simulink model "Loop_detailed_model_v12_bipolar"  (R2013a)
settings: Solver=ode3  SolverMode=SingleTasking  StartTime=0.0  StopTime=8e-3  FixedStep=FS/50  MaxStep=1e-4  RelTol=1e-3
InitFcn:
  | %%%%%%  set scope time range
  | T_STOP=str2num(get_param(gcs,'StopTime'));
  | if numel(T_STOP) > 1
  |    T_STOP=T_STOP(2);
  | else
  |    T_STOP=T_STOP(1);
  | end
  | T_STOP=num2str(T_STOP);
  | 
  | %%%%%%  set scope time range in system @init_callback_fct
  | T_STOP=num2str(str2num(get_param(gcs,'StopTime')));
  | 
  | childs = allchild(0);
  | sol=strfind(upper(get(allchild(0),'Tag')),'VIEWER_PARAMETERS');
  | 
  | if iscell(sol)
  |    ind=find(~cellfun(@isempty, strfind(upper(get(allchild(0),'Tag')),'VIEWER_PARAMETERS')));
  | else
  |    ind=sol;
  | end
  | %ind=find(~cellfun(@isempty, {strfind(upper(get(allchild(0),'Tag')),'VIEWER_PARAMETERS'),[]}))
  | if ~isempty(ind)
  |    for k=1:length(childs(ind))
  |       set_param(getfield(get(childs(ind(k)),'UserData'),'block'),'TimeRange', T_STOP);
  | %      get_param(getfield(get(childs(ind(k)),'UserData'),'block'),'TimeRange');
  | %    set_param(getfield(get(childs(ind),'UserData'),'block'),'TimeRange',T_STOP);
  | %    get_param(getfield(get(childs(ind),'UserData'),'block'),'TimeRange');
  |    end
  | else
  |     warning(sprintf('VIEWER_PARAMETERS object not found\nOpen the config dialog by hand for the first sim start'))
  | end
values from neighbouring files (symbols this model uses):
  FS = 5e-6    (= 5e-06)    [GalvoModel_v4_sys.m]    (also in GalvoModel_v6_sys.m = 5e-05; Galvo_process_analyze.m = 0.0001)
  Lc = 170e-6    (= 0.00017)    [GalvoModel_v6_sys.m]    (also in Galvo_process_analyze.m)
  Rc = 1.5    [GalvoModel_v6_sys.m]    (also in Galvo_process_analyze.m; frequenzgang_nichtinvert_opamp_koblitz_eas.m = 1)
  Rsh = 0.003    [GalvoModel_v6_sys.m]    (also in Galvo_sys_proto_v13_OFFSETS_MODEL_PT1B_proc.m = 0.075; frequenzgang_nichtinvert_opamp_koblitz_eas.m = 0.015)
  T1 = R1*C1    (= 0.000264)    [GalvoModel_v6_sys.m]
libraries: simulink x4
settings Model: BufferReuse=off  Creator=mainster  LastModifiedBy=mainster
settings SolverCC: AutoInsertRateTranBlk=on
settings OptimizationCC: InlineParams=on  BufferReuse=off
settings DebuggingCC: InitInArrayFormatMsg=none
settings HardwareCC: ProdLargestAtomicInteger=Long  ProdLargestAtomicFloat=Double  ProdEndianess=LittleEndian  ProdHWDeviceType=ARM Compatible->ARM Cortex

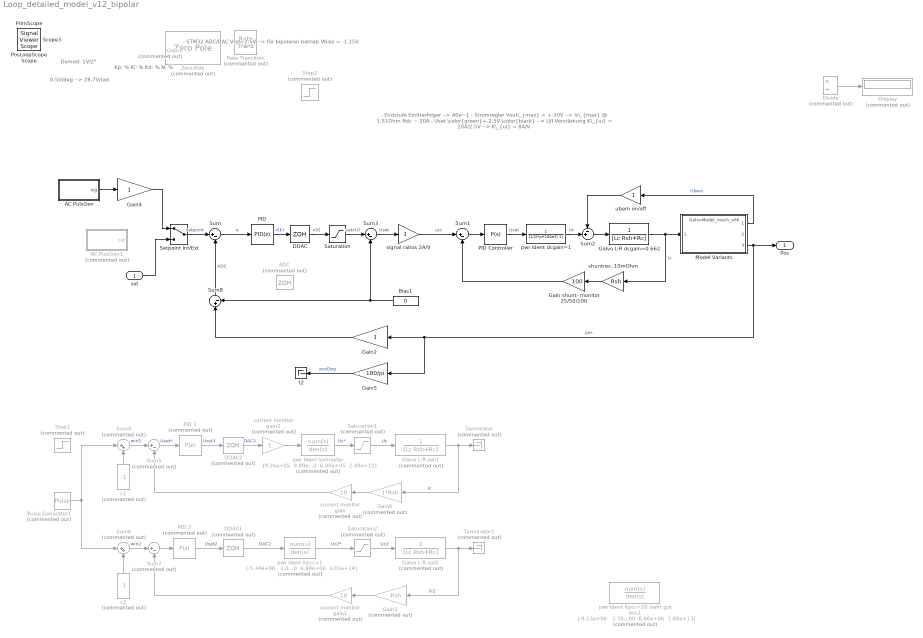
== system Loop_detailed_model_v12_bipolar ==
  note: - Endstufe Emitterfolger --> A0e~1
      | - Stromregler Vout\_{max} = +-30V
      |       --> Ic\_{max} @ 1.51Ohm Rdc ~ 20A
      | - Uset \color{green}+-2.5V \color{black}
      |       --> U/I Verstärkung K\_{ui} = 20A/2.5V
      |       --> K\_{ui} = 8A/V
  note: - STM32 ADC/DAC Vref=2.5V
      | --> für bipolaren betrieb Vbias = -1.25V
  note: Kp: % Ki: % Kd: % N: %
  note: 0.5V/deg --> 28.7V/rad
  note: Demod:
      | 1V/2°
  set : Inport
  AC PulsGen : Subsystem  mask{sigp=10, sigpp=0, offs=0}
      mask prompts: sigp "Insert signal peak"; sigpp "or signal peak-to-peak"; offs "Insert DC offset"
      mask TypeOptions sigp: PulsGen/Amplitude
      mask Callback sigp:
      | %sigp=get_param([gcb '/PulsGen'],'Amplitude')
      | %SigVal=2*sigp
      mask TypeOptions offs: offset/Value
      mask Display:
      | %str=sprintf('%s',get(gcbh,'ModelName'));
      | port_label('output', 1, '','texmode','off')
      | %text(.05,.98,['{\fontsize{12}\it\bf' strrep(str,'_',' ') '}'],'horizontalAlignment','left','verticalAlignment','top','texmode','on')
      | %text(.5,0.95,['{\fontsize{8}A_{peak}=}'],'horizontalAlignment','center','verticalAlignment','top','texmode','on')
      | disp(sprintf('Up=%.3g\nDC=%.3g',sigp, offs))
      | %disp(['Upp=' sigpp])%, offs))
      | %sprintf('sigpp==%s',sigpp)
      | %text(.15,.05,['{\fontsize{10}\itmechanics}'],'horizontalAlignment','left','verticalAlignment','bottom','texmode','on')
  AC PulsGen1 : Subsystem  Commented=on  mask{sigp=1, sigpp=0, offs=0}
      mask prompts: sigp "Insert signal peak"; sigpp "or signal peak-to-peak"; offs "Insert DC offset"
      mask TypeOptions sigp: PulsGen/Amplitude
      mask Callback sigp:
      | %sigp=get_param([gcb '/PulsGen'],'Amplitude')
      | %SigVal=2*sigp
      mask TypeOptions offs: offset/Value
      mask Display:
      | %str=sprintf('%s',get(gcbh,'ModelName'));
      | port_label('output', 1, '','texmode','off')
      | %text(.05,.98,['{\fontsize{12}\it\bf' strrep(str,'_',' ') '}'],'horizontalAlignment','left','verticalAlignment','top','texmode','on')
      | %text(.5,0.95,['{\fontsize{8}A_{peak}=}'],'horizontalAlignment','center','verticalAlignment','top','texmode','on')
      | disp(sprintf('Up=%.3g\nDC=%.3g',sigp, offs))
      | %disp(['Upp=' sigpp])%, offs))
      | %sprintf('sigpp==%s',sigpp)
      | %text(.15,.05,['{\fontsize{10}\itmechanics}'],'horizontalAlignment','left','verticalAlignment','bottom','texmode','on')
  ADC : ZeroOrderHold  Commented=on  SampleTime=FS
  Bias1 : Constant  Value=0  OutDataTypeStr=double  SampleTime=0
  DDAC : ZeroOrderHold  SampleTime=FS
      settings: AttributesFormatString=%<SampleTime>
  DDAC1 : ZeroOrderHold  Commented=on  SampleTime=FS
      settings: AttributesFormatString=%<SampleTime>
  DDAC2 : ZeroOrderHold  Commented=on  SampleTime=FS
      settings: AttributesFormatString=%<SampleTime>
  Display : Display  Commented=on
  Divide : Product  Commented=on  Inputs=*/
  Gain shunt- monitor 25/50/100 : Gain  Gain=100
  Gain1 : Gain  Commented=on  Gain=2
  Gain2 : Gain
  Gain3 : Gain  Commented=on  Gain=Rsh
  Gain4 : Gain  SampleTime=FS
  Gain5 : Gain  Gain=180/pi
  Gain6 : Gain  Commented=on  Gain=1*Rsh
  Galvo L-R dcgain=0.662 : TransferFcn  Numerator=1  Denominator=[Lc Rsh+Rc]
  Galvo L-R zeil1 : TransferFcn  Commented=on  Numerator=1  Denominator=[Lc Rsh+Rc]
  Galvo L-R zeil2 : TransferFcn  Commented=on  Numerator=1  Denominator=[Lc Rsh+Rc]
  Model Variants : ModelReference  ModelNameDialog=GalvoModel_mech_v60.slx  SimulationMode=Normal  ModelReferenceVersion=1.68  CopyOfModelName=GalvoModel_mech_v60.slx  DefaultDataLogging=on
      settings: AttributesFormatString=%<ActiveVariant>
  "PID " : simulink/Continuous/PID Controller  Controller=PID  TimeDomain=Discrete-time  SampleTime=FS  IntegratorMethod=Forward Euler  FilterMethod=Forward Euler  Form=Ideal  P=0.0159567680889438  I=1.35343300474195  D=0.0839511753460528  N=253.181387711443  InitialConditionSource=internal  InitialConditionForIntegrator=0  InitialConditionForFilter=0  ExternalReset=none  LimitOutput=off  UpperSaturationLimit=1.25  LowerSaturationLimit=-1.25  LinearizeAsGain=on  AntiWindupMode=clamping  Kb=1  TrackingMode=off  Kt=1  PParamMin=[]  PParamMax=[]  IParamMin=[]  IParamMax=[]  DParamMin=[]  DParamMax=[]  NParamMin=[]  NParamMax=[]  KbParamMin=[]  KbParamMax=[]  KtParamMin=[]  KtParamMax=[]  POutMin=[]  POutMax=[]  IOutMin=[]  IOutMax=[]  DOutMin=[]  DOutMax=[]  NOutMin=[]  NOutMax=[]  KbOutMin=[]  KbOutMax=[]  KtOutMin=[]  KtOutMax=[]  IntegratorOutMin=[]  IntegratorOutMax=[]  FilterOutMin=[]  FilterOutMax=[]  SumOutMin=[]  SumOutMax=[]  SumI1OutMin=[]  SumI1OutMax=[]  SumI2OutMin=[]  SumI2OutMax=[]  SumI3OutMin=[]  SumI3OutMax=[]  SumDOutMin=[]  SumDOutMax=[]  SaturationOutMin=[]  SaturationOutMax=[]  IntegratorContinuousStateAttributes=''  IntegratorStateMustResolveToSignalObject=off  IntegratorRTWStateStorageClass=Auto  FilterContinuousStateAttributes=''  FilterStateMustResolveToSignalObject=off  FilterRTWStateStorageClass=Auto
      settings: AttributesFormatString=UpLim=%<UpperSaturationLimit>\nLoLim=%<LowerSaturationLimit>\nKp=%<P>
  PID 1 : simulink/Continuous/PID Controller  Commented=on  Controller=P  TimeDomain=Discrete-time  SampleTime=FS  IntegratorMethod=Forward Euler  FilterMethod=Forward Euler  Form=Parallel  P=25.2263389172728  I=3745.38790742202  D=9.0248898483108e-05  N=10930.7783722874  InitialConditionSource=internal  InitialConditionForIntegrator=0  InitialConditionForFilter=0  ExternalReset=none  LimitOutput=off  UpperSaturationLimit=1.25  LowerSaturationLimit=-1.25  LinearizeAsGain=on  AntiWindupMode=clamping  Kb=1  TrackingMode=off  Kt=1  PParamMin=[]  PParamMax=[]  IParamMin=[]  IParamMax=[]  DParamMin=[]  DParamMax=[]  NParamMin=[]  NParamMax=[]  KbParamMin=[]  KbParamMax=[]  KtParamMin=[]  KtParamMax=[]  POutMin=[]  POutMax=[]  IOutMin=[]  IOutMax=[]  DOutMin=[]  DOutMax=[]  NOutMin=[]  NOutMax=[]  KbOutMin=[]  KbOutMax=[]  KtOutMin=[]  KtOutMax=[]  IntegratorOutMin=[]  IntegratorOutMax=[]  FilterOutMin=[]  FilterOutMax=[]  SumOutMin=[]  SumOutMax=[]  SumI1OutMin=[]  SumI1OutMax=[]  SumI2OutMin=[]  SumI2OutMax=[]  SumI3OutMin=[]  SumI3OutMax=[]  SumDOutMin=[]  SumDOutMax=[]  SaturationOutMin=[]  SaturationOutMax=[]  IntegratorContinuousStateAttributes=''  IntegratorStateMustResolveToSignalObject=off  IntegratorRTWStateStorageClass=Auto  FilterContinuousStateAttributes=''  FilterStateMustResolveToSignalObject=off  FilterRTWStateStorageClass=Auto
  PID 2 : simulink/Continuous/PID Controller  Commented=on  Controller=P  TimeDomain=Discrete-time  SampleTime=FS  IntegratorMethod=Forward Euler  FilterMethod=Forward Euler  Form=Parallel  P=9.78763876336799  I=3745.38790742202  D=9.0248898483108e-05  N=10930.7783722874  InitialConditionSource=internal  InitialConditionForIntegrator=0  InitialConditionForFilter=0  ExternalReset=none  LimitOutput=off  UpperSaturationLimit=1.25  LowerSaturationLimit=-1.25  LinearizeAsGain=on  AntiWindupMode=clamping  Kb=1  TrackingMode=off  Kt=1  PParamMin=[]  PParamMax=[]  IParamMin=[]  IParamMax=[]  DParamMin=[]  DParamMax=[]  NParamMin=[]  NParamMax=[]  KbParamMin=[]  KbParamMax=[]  KtParamMin=[]  KtParamMax=[]  POutMin=[]  POutMax=[]  IOutMin=[]  IOutMax=[]  DOutMin=[]  DOutMax=[]  NOutMin=[]  NOutMax=[]  KbOutMin=[]  KbOutMax=[]  KtOutMin=[]  KtOutMax=[]  IntegratorOutMin=[]  IntegratorOutMax=[]  FilterOutMin=[]  FilterOutMax=[]  SumOutMin=[]  SumOutMax=[]  SumI1OutMin=[]  SumI1OutMax=[]  SumI2OutMin=[]  SumI2OutMax=[]  SumI3OutMin=[]  SumI3OutMax=[]  SumDOutMin=[]  SumDOutMax=[]  SaturationOutMin=[]  SaturationOutMax=[]  IntegratorContinuousStateAttributes=''  IntegratorStateMustResolveToSignalObject=off  IntegratorRTWStateStorageClass=Auto  FilterContinuousStateAttributes=''  FilterStateMustResolveToSignalObject=off  FilterRTWStateStorageClass=Auto
  PID Controller : simulink/Continuous/PID Controller  Controller=P  TimeDomain=Continuous-time  SampleTime=1  IntegratorMethod=Forward Euler  FilterMethod=Forward Euler  Form=Ideal  P=0.980986879423172  I=31476.9869651078  D=0  N=100  InitialConditionSource=internal  InitialConditionForIntegrator=0  InitialConditionForFilter=0  ExternalReset=none  LimitOutput=off  UpperSaturationLimit=inf  LowerSaturationLimit=-inf  LinearizeAsGain=on  AntiWindupMode=none  Kb=1  TrackingMode=off  Kt=1  PParamMin=[]  PParamMax=[]  IParamMin=[]  IParamMax=[]  DParamMin=[]  DParamMax=[]  NParamMin=[]  NParamMax=[]  KbParamMin=[]  KbParamMax=[]  KtParamMin=[]  KtParamMax=[]  POutMin=[]  POutMax=[]  IOutMin=[]  IOutMax=[]  DOutMin=[]  DOutMax=[]  NOutMin=[]  NOutMax=[]  KbOutMin=[]  KbOutMax=[]  KtOutMin=[]  KtOutMax=[]  IntegratorOutMin=[]  IntegratorOutMax=[]  FilterOutMin=[]  FilterOutMax=[]  SumOutMin=[]  SumOutMax=[]  SumI1OutMin=[]  SumI1OutMax=[]  SumI2OutMin=[]  SumI2OutMax=[]  SumI3OutMin=[]  SumI3OutMax=[]  SumDOutMin=[]  SumDOutMax=[]  SaturationOutMin=[]  SaturationOutMax=[]  IntegratorContinuousStateAttributes=''  IntegratorStateMustResolveToSignalObject=off  IntegratorRTWStateStorageClass=Auto  FilterContinuousStateAttributes=''  FilterStateMustResolveToSignalObject=off  FilterRTWStateStorageClass=Auto
  Pulse Generator1 : DiscretePulseGenerator  Commented=on  PulseType=Time based  Amplitude=2  Period=4e-3  PulseWidth=50  SampleTime=FS
  Rate Transition : RateTransition  Commented=on  OutPortSampleTime=FS
  Saturation : Saturate  UpperLimit=125  LowerLimit=-125
      settings: AttributesFormatString=Up_lim=%<UpperLimit>\nLo_lim=%<LowerLimit>
  Saturation1 : Saturate  Commented=on  UpperLimit=30  LowerLimit=-30
      settings: AttributesFormatString=Up_lim=%<UpperLimit>\nLo_lim=%<LowerLimit>
  Saturation2 : Saturate  Commented=on  UpperLimit=30  LowerLimit=-30
      settings: AttributesFormatString=Up_lim=%<UpperLimit>\nLo_lim=%<LowerLimit>
  Setpoint Int/Ext : ManualSwitch  SampleTime=FS
  Step1 : Step  Commented=on  Time=2e-3  After=1.25  SampleTime=0
      settings: AttributesFormatString=Time:%<Time>\nAmp:%<After>
  Step2 : Step  Commented=on  Time=0  After=1.25  SampleTime=0
      settings: AttributesFormatString=Time:%<Time>\nAmp:%<After>
  Sum : Sum  Inputs=|+-  SampleTime=FS
  Sum1 : Sum  Inputs=|+-
  Sum2 : Sum  Inputs=-+|
  Sum3 : Sum  Inputs=|+-
  Sum4 : Sum  Commented=on  Inputs=|++  SampleTime=FS
  Sum5 : Sum  Commented=on  Inputs=|+-  SampleTime=FS
  Sum6 : Sum  Commented=on  Inputs=|++  SampleTime=FS
  Sum7 : Sum  Commented=on  Inputs=|+-  SampleTime=FS
  Sum8 : Sum  Inputs=|+-
  Terminator : Terminator  Commented=on
  Terminator1 : Terminator  Commented=on
  Zero-Pole : ZeroPole  Commented=on  Zeros=[]  Poles=[-1/T1 -1/T1]  Gain=(1/T1)^2
  c1 : Constant  Commented=on  Value=-1  SampleTime=FS
  c2 : Constant  Commented=on  Value=-1  SampleTime=FS
  current monitor gain : Gain  Commented=on  Gain=10
  current monitor gain1 : Gain  Commented=on  Gain=10
  current monitor gain2 : Gain  Commented=on
  "pwr Ident Kpcc=1 " : TransferFcn  Commented=on  Numerator="[-5.34e+06   3.00e+14]"  Denominator="[1.00e+00  6.89e+06  3.01e+14]"
  pwr Ident dcgain=1 : TransferFcn  Denominator=[1/(2*pi*100e3) 1]
  pwr Ident lochraster : TransferFcn  Commented=on  Numerator="[9.26e+05  9.89e+11]"  Denominator="[1.00e+00  6.00e+05  2.49e+12]"
  pwr Ident Kpcc=20 sieht gut aus1 : TransferFcn  Commented=on  Numerator="[-9.13e+06   3.76e+14]"  Denominator="[1.00e+00  6.60e+06  1.88e+13]"
  shuntres. 10mOhm : Gain  Gain=Rsh
  signal ratios 2A/V : Gain
  t2 : Terminator
  ubem on/off : Gain
  Pos : Outport  SampleTime=FS
  PosLoopScope : SignalViewerScope  IOType=viewer  NumInputPorts=5  LegendLocations=|  RefreshTime=0.035000
      | 0.75355     0.93607     0.18206    0.021763
      | 0.76421     0.72973      0.1714    0.038765
      | 0.79618     0.54149     0.13943    0.038765
      |  0.8175     0.36915     0.11812    0.021763
      | 0.68961      0.1809     0.16075    0.021763
      settings: ShowLegends=on  TimeRange=0.008  YMin=-10~-5~-20~-4~-5  YMax=10~5~20~4~20  SaveName=ScopeData2
  PrimScope : SignalViewerScope  IOType=viewer  NumInputPorts=6  LegendLocations=|  RefreshTime=0.054310
      | 0.72677     0.92301     0.16886    0.036879
      | 0.71487     0.76462     0.15898    0.036879
      | 0.77438     0.62345     0.10956    0.020704
      | 0.70296     0.44889     0.10956    0.020704
      | 0.78628     0.30771     0.11944    0.020704
      | 0.79818     0.14933     0.10956    0.020704
      settings: ShowLegends=on  TimeRange=0.008  YMin=-10~-5~-20~-4~-0.1~-20  YMax=10~5~20~4~0.4~20
  Scope : SignalViewerScope  IOType=viewer  RefreshTime=0.035000
  Scope3 : SignalViewerScope  IOType=viewer  ZoomMode=yonly  RefreshTime=0.035000
      settings: YMin=1  YMax=3  SaveName=ScopeData3
  wires:
  Sum/1 -> "PID "/1  "e"
  Galvo L-R dcgain=0.662/1 -> shuntres. 10mOhm/1, Model Variants/1  "Ic"
  "PID "/1 -> DDAC/1  "x(k)"
  PID Controller/1 -> pwr Ident dcgain=1/1  "Uset"
  pwr Ident dcgain=1/1 -> Sum2/2  "Uc"
  Saturation/1 -> Sum3/1  "satx(t)"
  Sum3/1 -> signal ratios 2A/V/1  "Uset"
  DDAC/1 -> Saturation/1  "x(t)"
  PID 1/1 -> DDAC2/1  "Uset3"
  pwr Ident lochraster/1 -> Saturation1/1  "Uc*"
  Galvo L-R zeil1/1 -> Gain6/1, Terminator/1  "Ic"
  Pulse Generator1/1 -> Sum6/1, Sum4/1
  c1/1 -> Sum4/2
  Sum4/1 -> Sum5/1  "win3"
  Sum5/1 -> PID 1/1  "Uset*"
  Saturation1/1 -> Galvo L-R zeil1/1  "Uc"
  Gain6/1 -> current monitor gain/1
  current monitor gain/1 -> Sum5/2
  PID 2/1 -> DDAC1/1  "Uset2"
  "pwr Ident Kpcc=1 "/1 -> Saturation2/1  "Uc2*"
  Galvo L-R zeil2/1 -> Gain3/1, Terminator1/1  "Ic2"
  c2/1 -> Sum6/2
  Sum6/1 -> Sum7/1  "win2"
  Sum7/1 -> PID 2/1
  Saturation2/1 -> Galvo L-R zeil2/1  "Uc2"
  Gain3/1 -> current monitor gain1/1
  current monitor gain1/1 -> Sum7/2
  DDAC1/1 -> "pwr Ident Kpcc=1 "/1  "DAC2"
  DDAC2/1 -> current monitor gain2/1  "DAC3"
  current monitor gain2/1 -> pwr Ident lochraster/1
  Sum8/1 -> Sum/2  "ADC"
  Bias1/1 -> Sum3/2, Sum8/2
  Setpoint Int/Ext/1 -> Sum/1  "setpoint"
  AC PulsGen/1(sig) -> Gain4/1
  Gain2/1 -> Sum8/1
  Sum1/1 -> PID Controller/1
  Gain shunt- monitor 25/50/100/1 -> Sum1/2
  shuntres. 10mOhm/1 -> Gain shunt- monitor 25/50/100/1
  signal ratios 2A/V/1 -> Sum1/1  "ucc"
  set/1 -> Setpoint Int/Ext/2
  Model Variants/3 -> Gain5/1, Gain2/1, Pos/1  "pos"
  Divide/1 -> Display/1
  Model Variants/1 -> ubem on/off/1  "Ubem"
  Sum2/1 -> Galvo L-R dcgain=0.662/1
  Gain4/1 -> Setpoint Int/Ext/1
  ubem on/off/1 -> Sum2/1
  Gain5/1 -> t2/1  "posDeg"

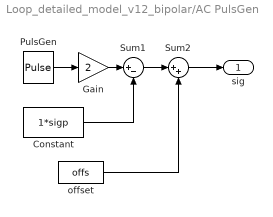
== system Loop_detailed_model_v12_bipolar/AC PulsGen ==
  Constant : Constant  Value=1*sigp
  Gain : Gain  Gain=2  SampleTime=FS
  PulsGen : DiscretePulseGenerator  PulseType=Time based  Amplitude=sigp  Period=4e-3  PulseWidth=50  PhaseDelay=0.5e-3  SampleTime=FS
      settings: AttributesFormatString=A=%<Amplitude>\nPeri=%<Period>
  Sum1 : Sum  Inputs=|+-  SampleTime=FS
  Sum2 : Sum  Inputs=|++  SampleTime=FS
  offset : Constant  Value=offs  SampleTime=FS
  sig : Outport
  wires:
  Sum2/1 -> sig/1
  PulsGen/1 -> Gain/1
  offset/1 -> Sum2/2
  Gain/1 -> Sum1/1
  Sum1/1 -> Sum2/1
  Constant/1 -> Sum1/2

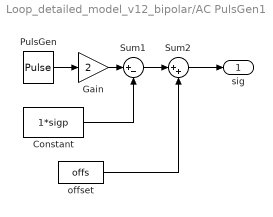
== system Loop_detailed_model_v12_bipolar/AC PulsGen1 ==
  Constant : Constant  Value=1*sigp
  Gain : Gain  Gain=2
  PulsGen : DiscretePulseGenerator  PulseType=Time based  Amplitude=sigp  Period=4e-3  PulseWidth=50  PhaseDelay=0.5e-3  SampleTime=FS
      settings: AttributesFormatString=A=%<Amplitude>\nPeri=%<Period>
  Sum1 : Sum  Inputs=|+-
  Sum2 : Sum  Inputs=|++
  offset : Constant  Value=offs
  sig : Outport
  wires:
  Sum2/1 -> sig/1
  PulsGen/1 -> Gain/1
  offset/1 -> Sum2/2
  Gain/1 -> Sum1/1
  Sum1/1 -> Sum2/1
  Constant/1 -> Sum1/2
